simulink model "qC_"  (R2020b)
settings: Solver=VariableStepAuto  StartTime=0.0  StopTime=10.0  RelTol=1e-3
values from neighbouring files (symbols this model uses):
  Bx = 0.0094    [q3.m]
  Jx = 0.000436    [q3.m]
  Ka = 1    [q2.m]    (also in q3.m)
  Ke = 1.59    [q2.m]    (also in q3.m)
  Kt = .49    (= 0.49)    [q2.m]    (also in q3.m)
  T = T * 0.001    (= 0.0001)    [q1.m]    (also in q2.m; q3.m)
libraries: cstblocks x2, simulink x1
settings Model: Creator=imhen  LastModifiedBy=Frienddo

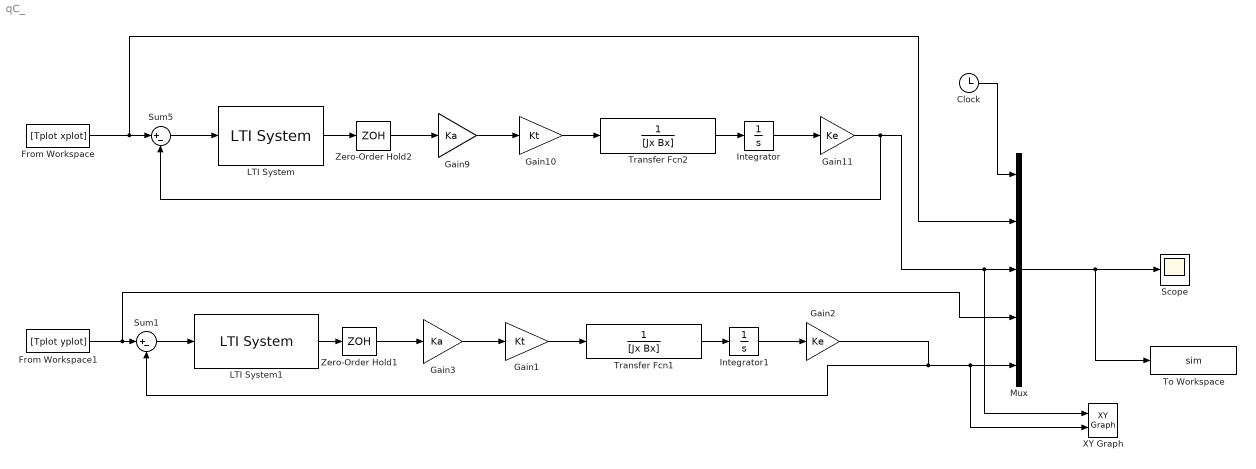
== system qC_ ==
  Clock : Clock
  From Workspace : FromWorkspace  VariableName=[Tplot xplot]
  From Workspace1 : FromWorkspace  VariableName=[Tplot yplot]
  Gain1 : Gain  Gain=Kt
  Gain10 : Gain  Gain=Kt
  Gain11 : Gain  Gain=Ke
  Gain2 : Gain  Gain=Ke
  Gain3 : Gain  Gain=Ka
  Gain9 : Gain  Gain=Ka
  Integrator : Integrator
  Integrator1 : Integrator
  LTI System : cstblocks/LTI System  sys=LLI_Lx_z  IC=[]
  LTI System1 : cstblocks/LTI System  sys=LLI_Ly_z  IC=[]
  Mux : Mux  Inputs=5
  Scope : Scope
  Sum1 : Sum  Inputs=|+-
  Sum5 : Sum  Inputs=|+-
  To Workspace : ToWorkspace  VariableName=sim  SaveFormat=Timeseries  SampleTime=-1
  Transfer Fcn1 : TransferFcn  Tag=TF1  Denominator=[Jx Bx]
  Transfer Fcn2 : TransferFcn  Tag=TF1  Denominator=[Jx Bx]
  XY Graph : simulink/Sinks/XY Graph  xmin=-1  xmax=170  ymin=-1  ymax=170  st=T
  Zero-Order Hold1 : ZeroOrderHold  SampleTime=T
  Zero-Order Hold2 : ZeroOrderHold  SampleTime=T
  wires:
  From Workspace/1 -> Mux/2, Sum5/1
  Sum5/1 -> LTI System/1
  LTI System/1 -> Zero-Order Hold2/1
  Zero-Order Hold2/1 -> Gain9/1
  Gain9/1 -> Gain10/1
  Gain10/1 -> Transfer Fcn2/1
  Transfer Fcn2/1 -> Integrator/1
  Integrator/1 -> Gain11/1
  Gain11/1 -> Sum5/2, XY Graph/1, Mux/3
  Clock/1 -> Mux/1
  Mux/1 -> To Workspace/1, Scope/1
  Sum1/1 -> LTI System1/1
  From Workspace1/1 -> Mux/4, Sum1/1
  LTI System1/1 -> Zero-Order Hold1/1
  Integrator1/1 -> Gain2/1
  Gain1/1 -> Transfer Fcn1/1
  Gain3/1 -> Gain1/1
  Zero-Order Hold1/1 -> Gain3/1
  Transfer Fcn1/1 -> Integrator1/1
  Gain2/1 -> XY Graph/2, Mux/5, Sum1/2
